simulink model "lab5_Odnofazn_Invertor_SimZakUpr"  (R2022a)
settings: Solver=ode23tb  StartTime=0.0  StopTime=0.5  MaxStep=1e-4  RelTol=1e-5
undefined symbols (not defined in the file): DCsource, RL, Sine_Wave, UB
libraries: spsFourierLib x4, spsGroundLib x3, spsCurrentMeasurementLib x2, spsSeriesRLCBranchLib x1, simulink x1, spsDCVoltageSourceLib x1, spsMultimeterLib x1, spsRMSLib x1, spsUniversalBridgeLib x1, spsVoltageMeasurementLib x1, spspowerguiLib x1
settings Model: Creator=79646  LastModifiedBy=админ

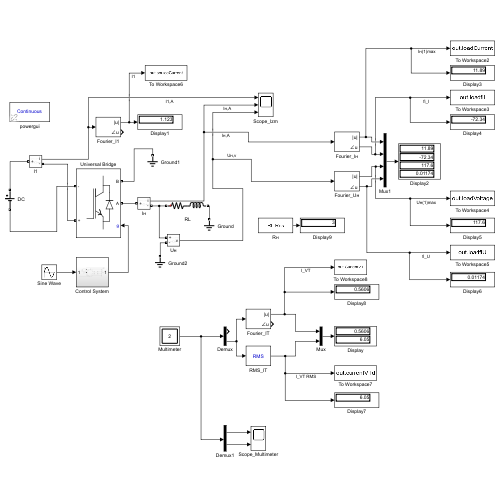
[thumbnail: Simulink's stored preview of the top-level diagram]
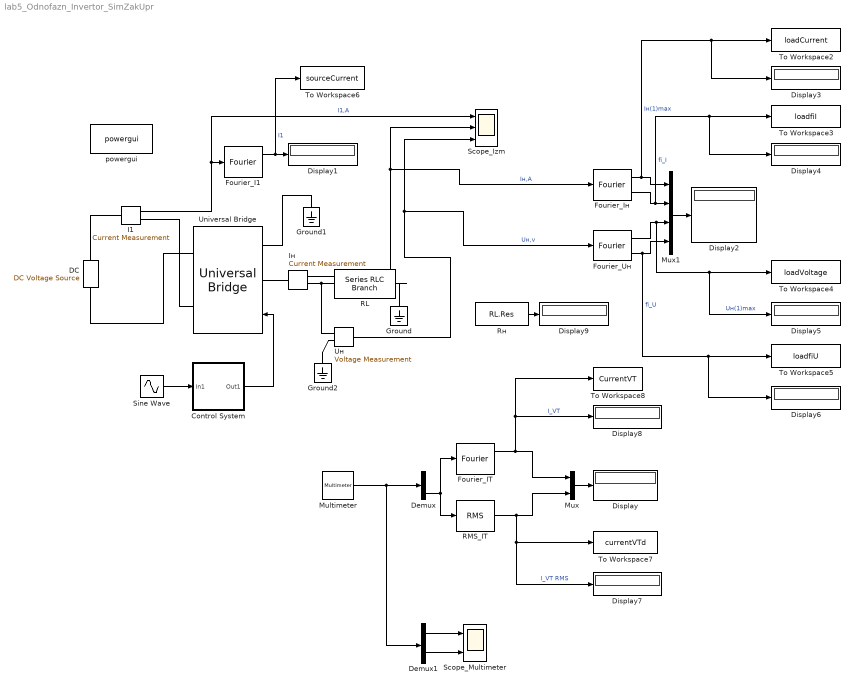
== system lab5_Odnofazn_Invertor_SimZakUpr ==
  " RL" : spsSeriesRLCBranchLib/Series RLC Branch  LConnTagsString=__new0  RConnTagsString=__new0  BranchType=RL  Resistance=RL.Res  Inductance=RL.Ind  SetiL0=off  InitialCurrent=0  Capacitance=1e-6  Setx0=off  InitialVoltage=0  Measurements=None
  Control System : Subsystem
  "DC  " : spsDCVoltageSourceLib/DC Voltage Source  Amplitude=DCsource.Voltage  Measurements=None
  Demux : Demux  Outputs=2
  Demux1 : Demux  Outputs=2
  Display{,1..9} (10 alike) : Display
  Fourier_I1 : spsFourierLib/Fourier  Freq=Fourier_I1IT.frec  n=Fourier_I1IT.harmonic  InInit=[0, 0]  Ts=0
      settings: SourceProductBaseCode=PS
  Fourier_IT : spsFourierLib/Fourier  Freq=Fourier_I1IT.frec  n=Fourier_I1IT.harmonic  InInit=[0, 0]  Ts=0
      settings: SourceProductBaseCode=PS
  Fourier_Iн : spsFourierLib/Fourier  Freq=Fourier_InUn.frec  n=Fourier_InUn.harmonic  InInit=[0, 0]  Ts=0
      settings: SourceProductBaseCode=PS
  Fourier_Uн : spsFourierLib/Fourier  Freq=Fourier_InUn.frec  n=Fourier_InUn.harmonic  InInit=[0, 0]  Ts=0
      settings: SourceProductBaseCode=PS
  Ground : spsGroundLib/Ground  LConnTagsString=a
  Ground1 : spsGroundLib/Ground  LConnTagsString=a
  Ground2 : spsGroundLib/Ground  LConnTagsString=a
  I1 : spsCurrentMeasurementLib/Current Measurement  PhasorSimulation=off  OutputType=Complex  PSBequivalent=0
  Iн : spsCurrentMeasurementLib/Current Measurement  PhasorSimulation=off  OutputType=Complex  PSBequivalent=0
  Multimeter : spsMultimeterLib/Multimeter  L=10  sel=[1 7]  yselected={}  Gain=[1 1]  OutputType=Complex  PlotAtSimulationStop=off  PhasorSimulation=off
  Mux : Mux  Inputs=2
  Mux1 : Mux
  RMS_IT : spsRMSLib/RMS  TrueRMS=on  Freq=RMS_T.frec  RMSInit=0  Ts=0
  Rн : Constant  Value=RL.Res
  Scope_Izm : Scope  NumInputPorts=3
  Scope_Multimeter : Scope  NumInputPorts=2
  Sine Wave : Sin  Amplitude=Sine_Wave.amplitude  Frequency=Sine_Wave.freq  Phase=Sine_Wave.Phase  SampleTime=0
  To Workspace2 : ToWorkspace  VariableName=loadCurrent  SampleTime=-1
      settings: Save2DSignal=2-D array (concatenate along first dimension)
  To Workspace3 : ToWorkspace  VariableName=loadfiI  SampleTime=-1
      settings: Save2DSignal=2-D array (concatenate along first dimension)
  To Workspace4 : ToWorkspace  VariableName=loadVoltage  SampleTime=-1
      settings: Save2DSignal=2-D array (concatenate along first dimension)
  To Workspace5 : ToWorkspace  VariableName=loadfiU  SampleTime=-1
      settings: Save2DSignal=2-D array (concatenate along first dimension)
  To Workspace6 : ToWorkspace  VariableName=sourceCurrent  SampleTime=-1
      settings: Save2DSignal=2-D array (concatenate along first dimension)
  To Workspace7 : ToWorkspace  VariableName=currentVTd  SampleTime=-1
      settings: Save2DSignal=2-D array (concatenate along first dimension)
  To Workspace8 : ToWorkspace  VariableName=CurrentVT  SampleTime=-1
      settings: Save2DSignal=2-D array (concatenate along first dimension)
  Universal Bridge : spsUniversalBridgeLib/Universal Bridge  Arms=2  SnubberResistance=UB.SnubberRs  SnubberCapacitance=UB.SnubberCs  Device=IGBT / Diodes  Ron=UB.R_on  Lon=0  ForwardVoltages="[UB.Vf  UB.Vfd]"  ForwardVoltage=0  GTOparameters=[ 10e-6 , 20e-6 ]  IGBTparameters=[ 1e-6 , 2e-6 ]  Measurements=All voltages and currents  Measurements_2=None  converterType=Rectifier
  Uн : spsVoltageMeasurementLib/Voltage Measurement  PhasorSimulation=off  OutputType=Complex  PSBequivalent=0
  powergui : spspowerguiLib/powergui  Priority=1  SimulationMode=Continuous  SampleTime=50e-6  frequency=60  Iterations=50  frequencyindice=0  Pbase=100e6  ErrMax=1e-4  UnitsV=kV  UnitsW=MW  buscounter=0  FunctionMessages=off  echomessages=off  EnableUseOfTLC=off  CurrentSourceSwitches=off  DisableSnubberDevices=off  DisableRonSwitches=off  DisableVfSwitches=off  DisplayEquations=off  AutomaticDiscreteSolvers=off  SolverType=Tustin/Backward Euler (TBE)  Interpol=off  ExternalGateDelay=off  methode=off  Ts=100  x0status=blocks  SPID=on  SwTol=0  HookPort=off  NonlinearTolerance=1e-4  nMaxIteration=100  ContinueOnMaxIteration=off  RestoreLinks=warning  ResistiveCurrentMeasurement=off  Frange=[0:2:500]  Ylog=off  Xlog=on  ShowGrid=off  save=off  variable=ZData  structure=0  ZoomFFT=off  StartTime=0.0  cycles=1  DisplayStyle=1  fundamental=60  FreqAxis=off  MaxFrequency=1000  frequencyindicesteady=1  RmsSteady=1  display=off
  wires:
  I1/1 -> Scope_Izm/1, Fourier_I1/1  "I1,A"
  Iн/1 -> Fourier_Iн/1, Scope_Izm/2  "Iн,А"
  Uн/1 -> Fourier_Uн/1, Scope_Izm/3  "Uн,v"
  Demux/2 -> Fourier_IT/1, RMS_IT/1
  RMS_IT/1 -> To Workspace7/1, Display7/1, Mux/2  "I_VT RMS"
  Fourier_IT/1 -> To Workspace8/1, Display8/1, Mux/1  "I_VT"
  Mux/1 -> Display/1
  Fourier_I1/1 -> To Workspace6/1, Display1/1  "I1"
  Fourier_Iн/1 -> To Workspace2/1, Display3/1, Mux1/1  "Iн(1)max"
  Fourier_Iн/2 -> To Workspace3/1, Display4/1, Mux1/2  "fi_I"
  Fourier_Uн/1 -> To Workspace4/1, Display5/1, Mux1/3  "Uн(1)max"
  Fourier_Uн/2 -> To Workspace5/1, Display6/1, Mux1/4  "fi_U"
  Mux1/1 -> Display2/1
  Sine Wave/1 -> Control System/1(In1)
  Control System/1(Out1) -> Universal Bridge/1
  Rн/1 -> Display9/1
  Demux1/1 -> Scope_Multimeter/1
  Demux1/2 -> Scope_Multimeter/2
  Multimeter/1 -> Demux1/1, Demux/1
  connections:
  "DC  "/RConn1 -- I1/LConn1
  I1/RConn1 -- Universal Bridge/RConn1
  "DC  "/LConn1 -- Universal Bridge/RConn2
  Iн/LConn1 -- Universal Bridge/LConn1
  " RL"/LConn1 -- Uн/LConn1 -- Iн/RConn1
  " RL"/RConn1 -- Ground/LConn1
  Universal Bridge/LConn2 -- Ground1/LConn1
  Ground2/LConn1 -- Uн/LConn2

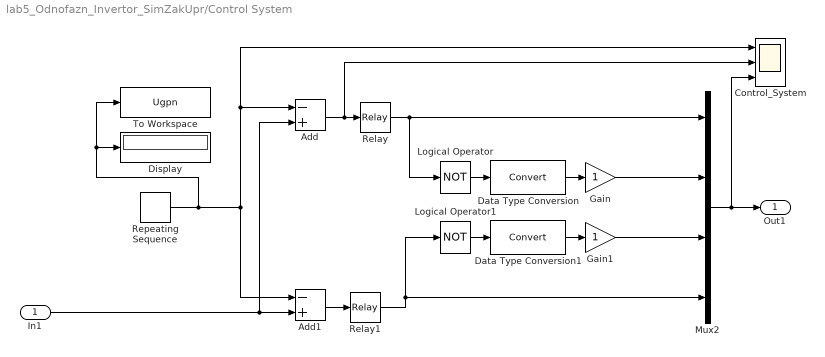
== system lab5_Odnofazn_Invertor_SimZakUpr/Control System ==
  In1 : Inport
  Add : Sum  Inputs=-+
  Add1 : Sum  Inputs=-+
  Control_System : Scope  NumInputPorts=3
  Data Type Conversion : DataTypeConversion  SaturateOnIntegerOverflow=off  RndMeth=Floor
  Data Type Conversion1 : DataTypeConversion  SaturateOnIntegerOverflow=off  RndMeth=Floor
  Display : Display
  Gain : Gain
  Gain1 : Gain
  Logical Operator : Logic  Operator=NOT  AllPortsSameDT=off  OutDataTypeStr=boolean
  Logical Operator1 : Logic  Operator=NOT  AllPortsSameDT=off  OutDataTypeStr=boolean
  Mux2 : Mux
  Relay : Relay
  Relay1 : Relay
  Repeating Sequence : simulink/Sources/Repeating Sequence  rep_seq_t=RepSec.Time  rep_seq_y=RepSec.Output
  To Workspace : ToWorkspace  VariableName=Ugpn  SampleTime=-1
      settings: Save2DSignal=2-D array (concatenate along first dimension)
  Out1 : Outport
  wires:
  Add1/1 -> Relay1/1
  Relay1/1 -> Logical Operator1/1, Mux2/4
  Relay/1 -> Logical Operator/1, Mux2/1
  Data Type Conversion1/1 -> Gain1/1
  In1/1 -> Add1/2, Add/2
  Data Type Conversion/1 -> Gain/1
  Logical Operator/1 -> Data Type Conversion/1
  Gain1/1 -> Mux2/3
  Repeating Sequence/1 -> Display/1, To Workspace/1, Add/1, Control_System/1, Add1/1
  Logical Operator1/1 -> Data Type Conversion1/1
  Gain/1 -> Mux2/2
  Add/1 -> Control_System/2, Relay/1
  Mux2/1 -> Control_System/3, Out1/1
